simulink model "circuitoRLCserie"  (Simulink 5.0)
settings: Solver=ode15s  StartTime=0.0  StopTime=0.08  RelTol=1e-3
values from neighbouring files (symbols this model uses):
  C = 100e-6    (= 0.0001)    [circuitoRLCserie_valores.m]
  L = 0.05    [circuitoRLCserie_valores.m]
  R = 5    [circuitoRLCserie_valores.m]
settings Model: LastModifiedBy=gaby

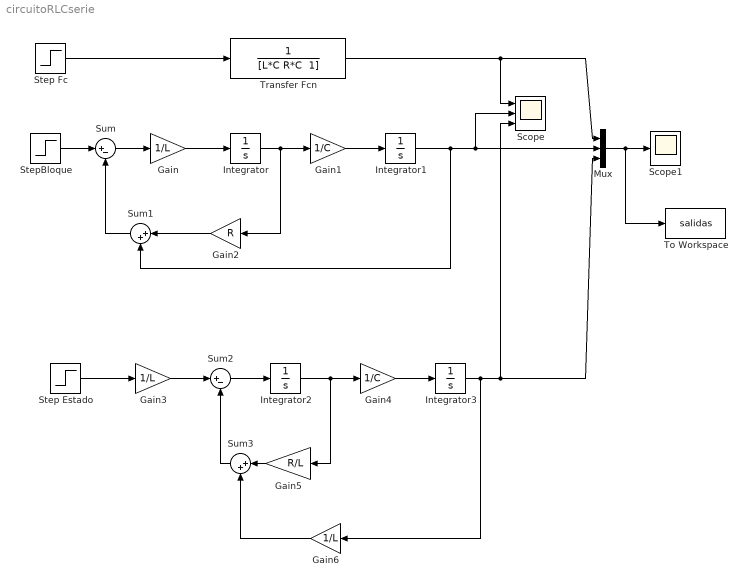
== system circuitoRLCserie ==
  Gain : Gain  Gain=1/L  SaturateOnIntegerOverflow=on
  Gain1 : Gain  Gain=1/C  SaturateOnIntegerOverflow=on
  Gain2 : Gain  Orientation=left  Gain=R  SaturateOnIntegerOverflow=on
  Gain3 : Gain  Gain=1/L  SaturateOnIntegerOverflow=on
  Gain4 : Gain  Gain=1/C  SaturateOnIntegerOverflow=on
  Gain5 : Gain  Orientation=left  Gain=R/L  SaturateOnIntegerOverflow=on
  Gain6 : Gain  Orientation=left  Gain=1/L  SaturateOnIntegerOverflow=on
  Integrator{,1..3} (4 alike) : Integrator
  Mux : Mux  Inputs=3
  Scope : Scope  NumInputPorts=3
      settings: YMin=-5~-5~-5  YMax=5~5~5
  Scope1 : Scope
  Step Estado : Step  Time=0.002  SampleTime=0
  Step Fc : Step  Time=0  SampleTime=0
  StepBloque : Step  Time=0.001  SampleTime=0
  Sum : Sum  Inputs=|+-  SaturateOnIntegerOverflow=on
  Sum1 : Sum  Orientation=left  Inputs=|++  SaturateOnIntegerOverflow=on
  Sum2 : Sum  Inputs=|+-  SaturateOnIntegerOverflow=on
  Sum3 : Sum  Orientation=left  Inputs=|++  SaturateOnIntegerOverflow=on
  To Workspace : ToWorkspace  VariableName=salidas  SampleTime=-1  SaveFormat=Array
  Transfer Fcn : TransferFcn  Denominator="[L*C R*C  1]"
  wires:
  Step Fc/1 -> Transfer Fcn/1
  Transfer Fcn/1 -> Scope/1, Mux/1
  Sum/1 -> Gain/1
  Gain/1 -> Integrator/1
  Integrator/1 -> Gain1/1, Gain2/1
  Gain1/1 -> Integrator1/1
  Gain2/1 -> Sum1/1
  Sum1/1 -> Sum/2
  Integrator1/1 -> Sum1/2, Scope/2, Mux/2
  StepBloque/1 -> Sum/1
  Step Estado/1 -> Gain3/1
  Gain3/1 -> Sum2/1
  Sum2/1 -> Integrator2/1
  Integrator2/1 -> Gain4/1, Gain5/1
  Gain4/1 -> Integrator3/1
  Gain5/1 -> Sum3/1
  Gain6/1 -> Sum3/2
  Sum3/1 -> Sum2/2
  Integrator3/1 -> Gain6/1, Scope/3, Mux/3
  Mux/1 -> Scope1/1, To Workspace/1
